simulink model "model_adp_TODO_2017b"  (R2017b)
settings: Solver=FixedStepAuto  StartTime=0.0  StopTime=3000  FixedStep=0.01  RelTol=1e-3
values from neighbouring files (symbols this model uses):
  f = [0 0 1 0 ... (first row only)    [Main.m]
  g = [0 0 ... (first row only)    [Main.m]
  q = diag([0.5 0.5 0.01 0.01])    [Main.m]
  r = diag([.01 .01])    [Main.m]
settings Model: Creator=Victus  LastModifiedBy=Victus
settings DataIOCC: ReturnWorkspaceOutputs=on
settings DebuggingCC: UnconnectedInputMsg=none  UnconnectedOutputMsg=none  UnconnectedLineMsg=none
settings ModelReferenceCC: EnableRefExpFcnMdlSchedulingChecks=off
settings SFSimCC: SimUseLocalCustomCode=on
settings RTWCC: Description=Generic Real-Time Target  RTWUseLocalCustomCode=on

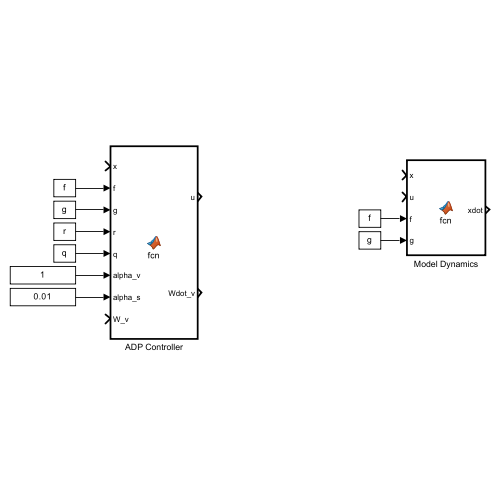
[thumbnail: Simulink's stored preview of the top-level diagram]
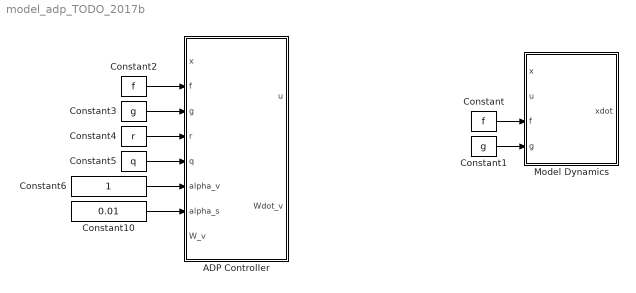
== system model_adp_TODO_2017b ==
  ADP Controller : MATLAB Function  TreatAsAtomicUnit=on
  Constant : Constant  Value=f
  Constant1 : Constant  Value=g
  Constant10 : Constant  Value=0.01
  Constant2 : Constant  Value=f
  Constant3 : Constant  Value=g
  Constant4 : Constant  Value=r
  Constant5 : Constant  Value=q
  Constant6 : Constant
  Model Dynamics : MATLAB Function  TreatAsAtomicUnit=on
  wires:
  Constant/1 -> Model Dynamics/3(f)
  Constant1/1 -> Model Dynamics/4(g)
  Constant3/1 -> ADP Controller/3(g)
  Constant2/1 -> ADP Controller/2(f)
  Constant4/1 -> ADP Controller/4(r)
  Constant5/1 -> ADP Controller/5(q)
  Constant6/1 -> ADP Controller/6(alpha_v)
  Constant10/1 -> ADP Controller/7(alpha_s)

== matlab function model_adp_TODO_2017b/ADP Controller ==
  data: x input; f input; g input; r input; q input; alpha_v input; alpha_s input; W_v input; u output; Wdot_v output
function [u, Wdot_v]= fcn(x, f, g, r, q, alpha_v, alpha_s, W_v)
x1 = x(1);
x2 = x(2);
x3 = x(3);
x4 = x(4);

%% Basis function
% mu_v = [x1^2; x1*x2; x1*x3; x1*x4;
%         x2^2; x2*x3; x2*x4;
%         x3^2; x3*x4;
%         x4^2]; %TODO: Experiment with other basis gunctions, such as RBF.
dmu_v = [2*x1    0     0     0;
           x2   x1     0     0;
           x3    0    x1     0;
           x4    0     0    x1;
           0  2*x2     0     0;
           0    x3    x2     0;
           0    x4     0    x2;
           0     0  2*x3     0;
           0     0    x4    x3;
           0     0     0  2*x4];

u = -1/2 * (r \ g') * dmu_v' * W_v;
Phi = dmu_v * (f*x + g*u);

%% Stabilizing term 
dJ_s = [x1 x2 x3 x4]';
if dJ_s' * (f*x+g*u) < 0
    Pi = 0;
else
    Pi = 1;
end
Delta = alpha_s * Pi * 1/2 * (dmu_v * g * (r \ g')) * dJ_s;

%% Update rule
e_c = x'*q*x + u'*r*u + Phi'*W_v;
Wdot_v = - alpha_v * Phi / (1 + Phi'*Phi)^2 * e_c + Delta;

== matlab function model_adp_TODO_2017b/Model Dynamics ==
  data: x input; u input; xdot output; f input; g input
function xdot = fcn(x,u,f,g)
    xdot = f*x + g*u;
end
